simulink model "zynqRadioFMStereoAD9361AD9364SL"  (R2016a)
settings: Solver=FixedStepDiscrete  SolverMode=SingleTasking  StartTime=0.0  StopTime=inf  RelTol=1e-3
PreLoadFcn:
  | stereoFMRxParams = getParamsFMExamplesAD9361AD9364;
InitFcn:
  | stereoFMRxParams = getParamsFMExamplesAD9361AD9364;
undefined symbols (not defined in the file or in its folder): F
libraries: simulink x1, dspsnks4 x1, commanabbnd3 x1, sdrzblksprivate x1, zc706fmc234_lib x1
CloseFcn:
  | clear stereoFMRxParams
Description:
  | This model uses Zynq-based SDR hardware with Analog Devices(TM) FMCOMMS2, FMCOMMS3 or FMCOMMS4 to perform FM stereo demodulation using Simulink(R).
settings Model: SimulationMode=accelerator  Creator=The MathWorks, Inc.  LastModifiedBy=The MathWorks, Inc.
settings DataIOCC: SaveFormat=Structure  SaveOutput=off  SignalLogging=off  DSMLogging=off  SaveTime=off
settings OptimizationCC: ExpressionDepthLimit=2147483647  EfficientMapNaN2IntZero=off  SimCompilerOptimization=on
settings DebuggingCC: UnderspecifiedInitializationDetection=Classic  MergeDetectMultiDrivingBlocksExec=none  SolverPrmCheckMsg=warning  InheritedTsInSrcMsg=none  MultiTaskCondExecSysMsg=none  ParameterPrecisionLossMsg=none  FcnCallInpInsideContextMsg=UseLocalSettings  AllowSymbolicDim=off  StateNameClashWarn=warning
settings HardwareCC: ProdBitPerPointer=32  ProdLargestAtomicFloat=None  ProdIntDivRoundTo=Undefined  ProdEndianess=Unspecified  ProdWordSize=32  ProdHWDeviceType=32-bit Generic  TargetBitPerPointer=64  TargetLongLongMode=on  TargetIntDivRoundTo=Zero  TargetEndianess=LittleEndian  TargetWordSize=64  TargetHWDeviceType=Generic->MATLAB Host Computer  ProdEqTarget=off
settings ModelReferenceCC: PropagateSignalLabelsOutOfModel=off
settings SFSimCC: SimIntegrity=off
settings RTWCC: CustomSourceCode=|
  | #include <stdio.h>
  | #include <stdlib.h>
settings CodeAppCC: MaxIdLength=128
settings GRTTargetCC: CombineOutputUpdateFcns=off  GRTInterface=on
settings ConfigComp: CovModelRefEnable=Off  CovSFcnEnable=off

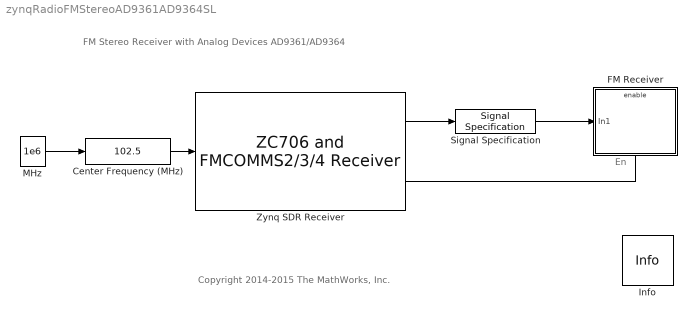
== system zynqRadioFMStereoAD9361AD9364SL ==
  note: En
  note: Copyright 2014-2015 The MathWorks, Inc.
  note: FM Stereo Receiver with Analog Devices AD9361/AD9364
  Center Frequency (MHz) : simulink/Math Operations/Slider Gain  low=87.5  gain=102.5  high=108
  FM Receiver : Subsystem  TreatAsAtomicUnit=on
      mask Display:
      | plot(0,0,100,100,[5+4.5*[0:.15:10] 50 50 50 50+4.5*[0:10]],[85+10*[sin([0:.15:10]*pi*2+cumsum(sin([0:.15:10]*pi/5))/2)] 85 99 75   10*sin([0:10]*pi/5)+85])
      | disp('\nFM\nBroadcast\nDemodulator')
  Info : sdrzblksprivate/Info  SystemSampleTime=-1
  MHz : Constant  Value=1e6  VectorParams1D=off  SampleTime=stereoFMRxParams.RadioFrameLength/stereoFMRxParams.RadioSampleRate  FramePeriod=-1
  Signal Specification : SignalSpecification  SampleTime=stereoFMRxParams.RadioFrameLength/stereoFMRxParams.RadioSampleRate
  Zynq SDR Receiver : zc706fmc234_lib/ZC706 and  FMCOMMS2//3//4  Receiver  IPAddress=192.168.3.2  CenterFrequencySource=Input port  CenterFrequency=2400000000  GainSource=AGC Fast Attack  Gain=1  ChannelMapping=1  BasebandSampleRate=stereoFMRxParams.RadioSampleRate  EnableBurstMode=off  NumFramesInBurst=20  OutputDataType=single  SamplesPerFrame=stereoFMRxParams.RadioFrameLength  LostSamplesOutputPort=off  RSSIOutputPort=off  DMATimeoutValue=1  blockMode=Normal  EnableQuadratureTracking=on  EnableRFDCTracking=on  EnableBasebandDCTracking=on  BypassUserLogic=on  ShowAdvancedProperties=on  ShowInternalProperties=off  subDeviceList=zynqReceiver  sdrExecutionMode=HW  dataUDPPort=-1  ctrlUDPPort=-1  SourceSelect=RF data  SourceConfiguration1=1023  FIRCoefficientSize=[ 128; 128 ]  FIRCoefficients=[ 111, -87, 147, -127, -18, -286, -312, -555, -601, -722, -642, -555, -303, -66, 221, 393, 488, 403, 219, -74, -343, -550, -582, -450, -146, 221, 569, 759, 735, 463, 20, -487, -885, -1048, -883, -418, 243, 897, 1340, 1394, 1002, 228, -715, -1549, -1980, -1819, -1028, 217, 1583, 2635, 2980, 2377, 853, -1275, -3435, -4926, -5080, -3454, 40, 5065, 10903, 16581, 21085, 23573, 23573, 21085, 16581, 10903, 5065, 40, -3454, -5080, -4926, -3435, -1275, 853, 2377, 2980, 2635, 1583, 217, -1028, -1819, -1980, -1549, -715, 228, 1002, 1394, 1340, 897, 243, -418, -883, -1048, -885, -487, 20, 463, 735, 759, 569, 221, -146, -450, -582, -550, -343, -74, 219, 403, 488, 393, 221, -66, -303, -555, -642, -722, -601, -555, -312, -286, -18, -127, 147, -87, 111; 382, -200, 711, -41, 645, 36, 346, -194, -119, -543, -472, -646, -404, -312, 45, 197, 413, 346, 241, -93, -373, -680, -755, -689, -356, 51, 515, 795, 870, 609, 136, -488, -1009, -1303, -1191, -712, 69, 885, 1516, 1692, 1336, 468, -662, -1740, -2378, -2329, -1494, -55, 1620, 2995, 3584, 3045, 1368, -1121, -3755, -5708, -6156, -4542, -710, 4969, 11669, 18243, 23486, 26391, 26391, 23486, 18243, 11669, 4969, -710, -4542, -6156, -5708, -3755, -1121, 1368, 3045, 3584, 2995, 1620, -55, -1494, -2329, -2378, -1740, -662, 468, 1336, 1692, 1516, 885, 69, -712, -1191, -1303, -1009, -488, 136, 609, 870, 795, 515, 51, -356, -689, -755, -680, -373, -93, 241, 346, 413, 197, 45, -312, -404, -646, -472, -543, -119, -194, 346, 36, 645, -41, 711, -200, 382 ]  FIRGain=[ 0; -12 ]  FIRDecimInterpFactor=[ 4; 4 ]  AnalogFilterCutoff=[ 2560000; 2560000 ]  FilterPathRates=[ 737280000, 184320000, 61440000, 30720000, 15360000, 3840000; 737280000, 184320000, 61440000, 30720000, 15360000, 3840000 ]  FilterDesignTypeForTx=DefaultFilterFromOther  FilterDesignTypeForRx=DefaultFilter  BISTLoopbackConfig=No Loopback  BISTPRBSMode=PRBS Disable  BISTToneMode=Tone Disable  BISTToneFrequency=F/32  BISTToneLevel=-6  BISTChannelMask=0  DataIsComplex=on  SimulateUsing=Code generation
  wires:
  Zynq SDR Receiver/2 -> FM Receiver/Enable
  MHz/1 -> Center Frequency (MHz)/1
  Center Frequency (MHz)/1 -> Zynq SDR Receiver/1
  Zynq SDR Receiver/1 -> Signal Specification/1
  Signal Specification/1 -> FM Receiver/1(In1)

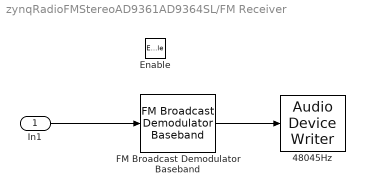
== system zynqRadioFMStereoAD9361AD9364SL/FM Receiver ==
  In1 : Inport
  Enable : EnablePort
  48045Hz : dspsnks4/Audio Device Writer  Driver=DirectSound  Device=Default  InheritSampleRate=on  SampleRate=44100  BitDepth=16-bit integer  BufferSize=4096  NumBuffers=10  DefaultOutputChannelMapping=on  OutputChannelMapping=1:2  OutputNumUnderrunSamples=off  DriverIdx=1  DeviceWarnFlag=''
  FM Broadcast Demodulator Baseband : commanabbnd3/FM Broadcast Demodulator Baseband  SampleRate=stereoFMRxParams.RadioSampleRate  FrequencyDeviation=stereoFMRxParams.FrequencyDeviation  FilterTimeConstant=stereoFMRxParams.FilterTimeConstant  AudioSampleRate=stereoFMRxParams.AudioSampleRate  PlaySound=off  BufferSize=stereoFMRxParams.BufferSize  Stereo=on  SimulateUsing=Code generation
  wires:
  In1/1 -> FM Broadcast Demodulator Baseband/1
  FM Broadcast Demodulator Baseband/1 -> 48045Hz/1
